simulink model "ThermalMon"  (R2023b)
settings: Solver=FixedStepAuto  StartTime=0.0  StopTime=10.0  RelTol=1e-3
undefined symbols (not defined in the file): THERMALMON_FILTER_ALPHA, THERMALMON_T_CRITICAL_TH, THERMALMON_T_OVERHEAT_TH, THERMALMON_T_UNDER_TH, THERMALMON_T_WARNING_TH, THERMALMON_TS_SEC, ThermalState_e
libraries: simulink x10
settings Model: DataDictionary=ThermalMon.sldd  Creator=84339  LastModifiedBy=84339
settings OptimizationCC: DefaultParameterBehavior=Inlined  EnhancedBackFolding=on  PassReuseOutputArgsAs=Individual arguments  ZeroExternalMemoryAtStartup=off  ZeroInternalMemoryAtStartup=off  OptimizeBlockOrder=speed  DifferentSizesBufferReuse=on  OptimizationCustomize=off  EfficientTunableParamExpr=on
settings DebuggingCC: ParameterTunabilityLossMsg=error
settings ModelReferenceCC: ModelReferenceNumInstancesAllowed=Single
settings SFSimCC: MATLABDynamicMemAlloc=off
settings RTWCC: Description=Embedded Coder  SystemTargetFile=ert.tlc  EmbeddedCoderDictionary=ASW.sldd  GenCodeOnly=on  TemplateMakefile=ert_default_tmf  DataTypeReplacement=CDataTypesFixedWidth
settings CodeAppCC: ForceParamTrailComments=on  IgnoreCustomStorageClasses=off  OperatorAnnotations=on  SimulinkDataObjDesc=on  SFDataObjDesc=on  InsertBlockDesc=on
settings ERTTargetCC: TargetLangStandard=C99 (ISO)  GenerateSampleERTMain=on  InlinedParameterPlacement=NonHierarchical  ERTCustomFileTemplate=example_file_process.tlc  MaxIdInt64=INT64_MAX  MinIdInt64=INT64_MIN  MaxIdUint64=UINT64_MAX  MaxIdInt32=INT32_MAX  MinIdInt32=INT32_MIN  MaxIdUint32=UINT32_MAX  MaxIdInt16=INT16_MAX  MinIdInt16=INT16_MIN  MaxIdUint16=UINT16_MAX  MaxIdInt8=INT8_MAX  MinIdInt8=INT8_MIN  MaxIdUint8=UINT8_MAX

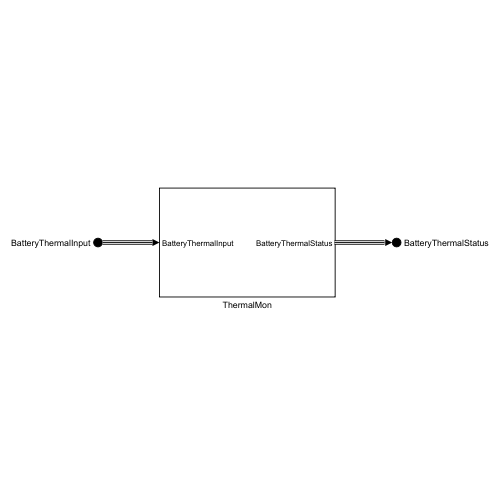
[thumbnail: Simulink's stored preview of the top-level diagram]
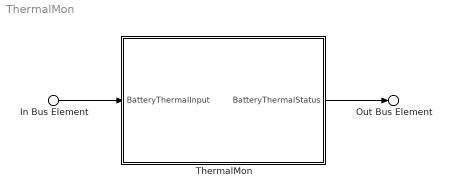
== system ThermalMon ==
  In Bus Element : Inport  PortName=BatteryThermalInput
  ThermalMon : Subsystem
      settings: RTWFcnNameOpts=Use subsystem name
  Out Bus Element : Outport  PortName=BatteryThermalStatus
  wires:
  In Bus Element/1 -> ThermalMon/1(BatteryThermalInput)
  ThermalMon/1(BatteryThermalStatus) -> Out Bus Element/1

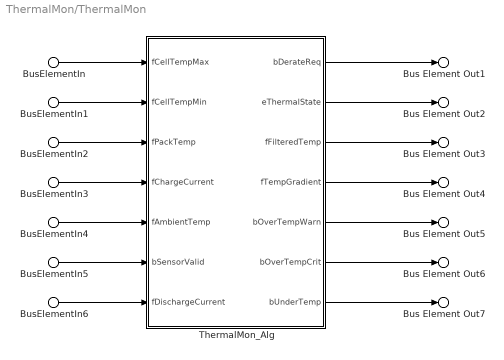
== system ThermalMon/ThermalMon ==
  BusElementIn : Inport  PortName=BatteryThermalInput  Element=fCellTempMax
  BusElementIn1 : Inport  PortName=BatteryThermalInput  Element=fCellTempMin
  BusElementIn2 : Inport  PortName=BatteryThermalInput  Element=fPackTemp
  BusElementIn3 : Inport  PortName=BatteryThermalInput  Element=fChargeCurrent
  BusElementIn4 : Inport  PortName=BatteryThermalInput  Element=fAmbientTemp
  BusElementIn5 : Inport  PortName=BatteryThermalInput  Element=bSensorValid
  BusElementIn6 : Inport  PortName=BatteryThermalInput  Element=fDischargeCurrent
  ThermalMon_Alg : Subsystem
      settings: RTWFcnNameOpts=Use subsystem name
  Bus Element Out2 : Outport  PortName=BatteryThermalStatus  Element=eThermalState
  Bus Element Out3 : Outport  PortName=BatteryThermalStatus  Element=fFilteredTemp
  Bus Element Out4 : Outport  PortName=BatteryThermalStatus  Element=fTempGradient
  Bus Element Out5 : Outport  PortName=BatteryThermalStatus  Element=bOverTempWarn
  Bus Element Out6 : Outport  PortName=BatteryThermalStatus  Element=bOverTempCrit
  Bus Element Out1 : Outport  PortName=BatteryThermalStatus  Element=bDerateReq
  Bus Element Out7 : Outport  PortName=BatteryThermalStatus  Element=bUnderTemp
  wires:
  BusElementIn/1 -> ThermalMon_Alg/1(fCellTempMax)
  BusElementIn1/1 -> ThermalMon_Alg/2(fCellTempMin)
  ThermalMon_Alg/1(bDerateReq) -> Bus Element Out1/1
  ThermalMon_Alg/2(eThermalState) -> Bus Element Out2/1
  ThermalMon_Alg/3(fFilteredTemp) -> Bus Element Out3/1
  ThermalMon_Alg/4(fTempGradient) -> Bus Element Out4/1
  ThermalMon_Alg/5(bOverTempWarn) -> Bus Element Out5/1
  ThermalMon_Alg/6(bOverTempCrit) -> Bus Element Out6/1
  BusElementIn6/1 -> ThermalMon_Alg/7(fDischargeCurrent)
  BusElementIn2/1 -> ThermalMon_Alg/3(fPackTemp)
  BusElementIn3/1 -> ThermalMon_Alg/4(fChargeCurrent)
  BusElementIn4/1 -> ThermalMon_Alg/5(fAmbientTemp)
  BusElementIn5/1 -> ThermalMon_Alg/6(bSensorValid)
  ThermalMon_Alg/7(bUnderTemp) -> Bus Element Out7/1

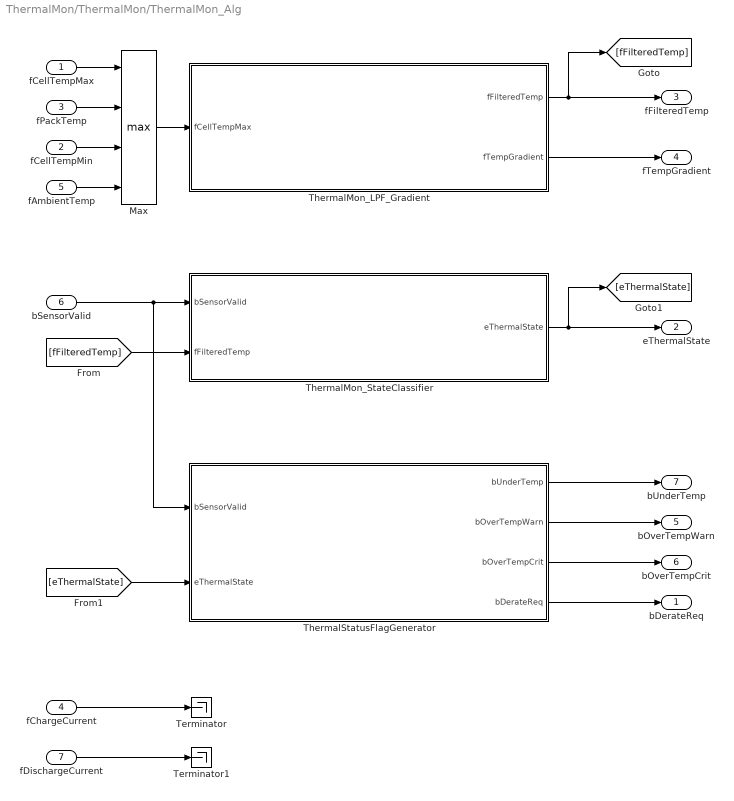
== system ThermalMon/ThermalMon/ThermalMon_Alg ==
  fCellTempMax : Inport  OutDataTypeStr=single
  fCellTempMin : Inport  Port=2  OutDataTypeStr=single
  fPackTemp : Inport  Port=3  OutDataTypeStr=single
  fChargeCurrent : Inport  Port=4  OutDataTypeStr=single
  fAmbientTemp : Inport  Port=5  OutDataTypeStr=single
  bSensorValid : Inport  Port=6  OutDataTypeStr=boolean
  fDischargeCurrent : Inport  Port=7  OutDataTypeStr=single
  Max : MinMax  Function=max  Inputs=4  OutDataTypeStr=single
  Terminator : Terminator
  Terminator1 : Terminator
  ThermalMon_LPF_Gradient : Subsystem  TreatAsAtomicUnit=on
      settings: RTWSystemCode=Nonreusable function  RTWFcnNameOpts=Use subsystem name
  ThermalMon_StateClassifier : Subsystem  TreatAsAtomicUnit=on
      settings: RTWSystemCode=Nonreusable function  RTWFcnNameOpts=Use subsystem name
  ThermalStatusFlagGenerator : Subsystem  TreatAsAtomicUnit=on
      settings: RTWSystemCode=Nonreusable function  RTWFcnNameOpts=Use subsystem name
  bDerateReq : Outport  OutDataTypeStr=boolean
  eThermalState : Outport  Port=2  OutDataTypeStr=Enum: ThermalState_e
  fFilteredTemp : Outport  Port=3  OutDataTypeStr=single
  fTempGradient : Outport  Port=4  OutDataTypeStr=single
  bOverTempWarn : Outport  Port=5  OutDataTypeStr=boolean
  bOverTempCrit : Outport  Port=6  OutDataTypeStr=boolean
  bUnderTemp : Outport  Port=7  OutDataTypeStr=boolean
  wires:
  [fFilteredTemp] -> ThermalMon_StateClassifier/2(fFilteredTemp)
  fPackTemp/1 -> Max/2
  ThermalMon_LPF_Gradient/1(fFilteredTemp) -> fFilteredTemp/1, [fFilteredTemp]
  bSensorValid/1 -> ThermalStatusFlagGenerator/1(bSensorValid), ThermalMon_StateClassifier/1(bSensorValid)
  Max/1 -> ThermalMon_LPF_Gradient/1(fCellTempMax)
  ThermalMon_LPF_Gradient/2(fTempGradient) -> fTempGradient/1
  [eThermalState] -> ThermalStatusFlagGenerator/2(eThermalState)
  fDischargeCurrent/1 -> Terminator1/1
  fChargeCurrent/1 -> Terminator/1
  ThermalStatusFlagGenerator/1(bUnderTemp) -> bUnderTemp/1
  ThermalStatusFlagGenerator/3(bOverTempCrit) -> bOverTempCrit/1
  ThermalStatusFlagGenerator/4(bDerateReq) -> bDerateReq/1
  fCellTempMax/1 -> Max/1
  fCellTempMin/1 -> Max/3
  ThermalMon_StateClassifier/1(eThermalState) -> [eThermalState], eThermalState/1
  fAmbientTemp/1 -> Max/4
  ThermalStatusFlagGenerator/2(bOverTempWarn) -> bOverTempWarn/1

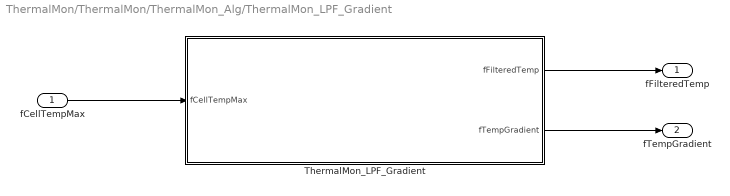
== system ThermalMon/ThermalMon/ThermalMon_Alg/ThermalMon_LPF_Gradient ==
  fCellTempMax : Inport
  ThermalMon_LPF_Gradient : MATLAB Function  TreatAsAtomicUnit=on
  fFilteredTemp : Outport
  fTempGradient : Outport  Port=2
  wires:
  fCellTempMax/1 -> ThermalMon_LPF_Gradient/1(fCellTempMax)
  ThermalMon_LPF_Gradient/1(fFilteredTemp) -> fFilteredTemp/1
  ThermalMon_LPF_Gradient/2(fTempGradient) -> fTempGradient/1

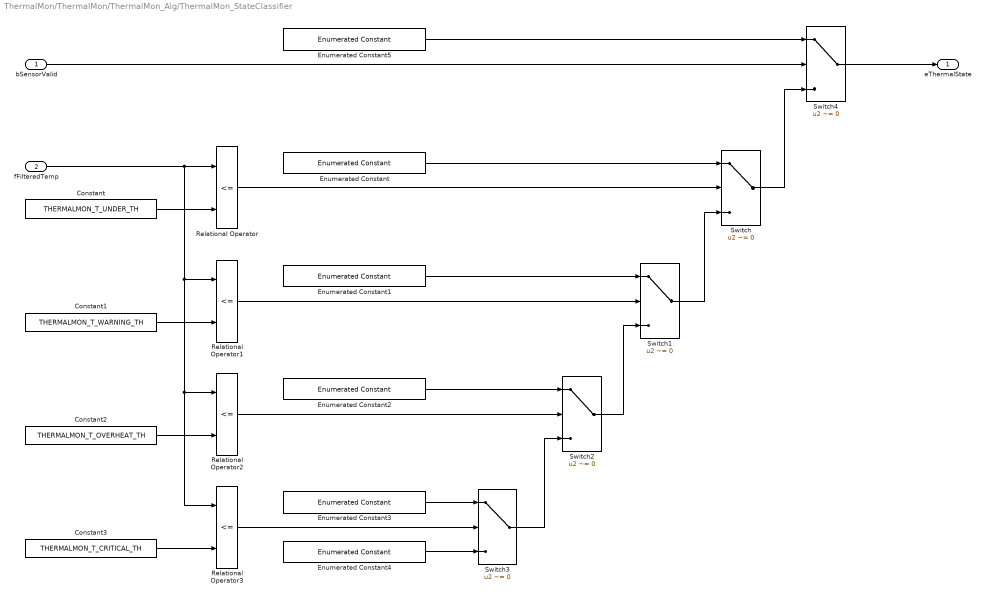
== system ThermalMon/ThermalMon/ThermalMon_Alg/ThermalMon_StateClassifier ==
  bSensorValid : Inport
  fFilteredTemp : Inport  Port=2
  Constant : Constant  Value=THERMALMON_T_UNDER_TH
  Constant1 : Constant  Value=THERMALMON_T_WARNING_TH
  Constant2 : Constant  Value=THERMALMON_T_OVERHEAT_TH
  Constant3 : Constant  Value=THERMALMON_T_CRITICAL_TH
  Enumerated Constant : simulink/Sources/Enumerated Constant  OutDataTypeStr=Enum: ThermalState_e  Value=ThermalState_e.THERM_UNDER_TEMP  SampleTime=inf
  Enumerated Constant1 : simulink/Sources/Enumerated Constant  OutDataTypeStr=Enum: ThermalState_e  Value=ThermalState_e.THERM_NORMAL  SampleTime=inf
  Enumerated Constant2 : simulink/Sources/Enumerated Constant  OutDataTypeStr=Enum: ThermalState_e  Value=ThermalState_e.THERM_WARNING  SampleTime=inf
  Enumerated Constant3 : simulink/Sources/Enumerated Constant  OutDataTypeStr=Enum: ThermalState_e  Value=ThermalState_e.THERM_OVERHEAT  SampleTime=inf
  Enumerated Constant4 : simulink/Sources/Enumerated Constant  OutDataTypeStr=Enum: ThermalState_e  Value=ThermalState_e.THERM_CRITICAL  SampleTime=inf
  Enumerated Constant5 : simulink/Sources/Enumerated Constant  OutDataTypeStr=Enum: ThermalState_e  Value=ThermalState_e.THERM_CRITICAL  SampleTime=inf
  Relational Operator{,1..3} (4 alike) : RelationalOperator  Operator=<=  OutDataTypeStr=boolean  RndMeth=Simplest  InputSameDT=off
  Switch{,1..4} (5 alike) : Switch  Criteria=u2 ~= 0  SaturateOnIntegerOverflow=off  InputSameDT=off
  eThermalState : Outport
  wires:
  Relational Operator/1 -> Switch/2
  Constant/1 -> Relational Operator/2
  Enumerated Constant/1 -> Switch/1
  Relational Operator1/1 -> Switch1/2
  Constant1/1 -> Relational Operator1/2
  Enumerated Constant1/1 -> Switch1/1
  Constant2/1 -> Relational Operator2/2
  Enumerated Constant2/1 -> Switch2/1
  Relational Operator2/1 -> Switch2/2
  Relational Operator3/1 -> Switch3/2
  Enumerated Constant3/1 -> Switch3/1
  Constant3/1 -> Relational Operator3/2
  fFilteredTemp/1 -> Relational Operator/1, Relational Operator1/1, Relational Operator2/1, Relational Operator3/1
  Enumerated Constant4/1 -> Switch3/3
  Switch1/1 -> Switch/3
  Switch3/1 -> Switch2/3
  Switch2/1 -> Switch1/3
  bSensorValid/1 -> Switch4/2
  Enumerated Constant5/1 -> Switch4/1
  Switch/1 -> Switch4/3
  Switch4/1 -> eThermalState/1

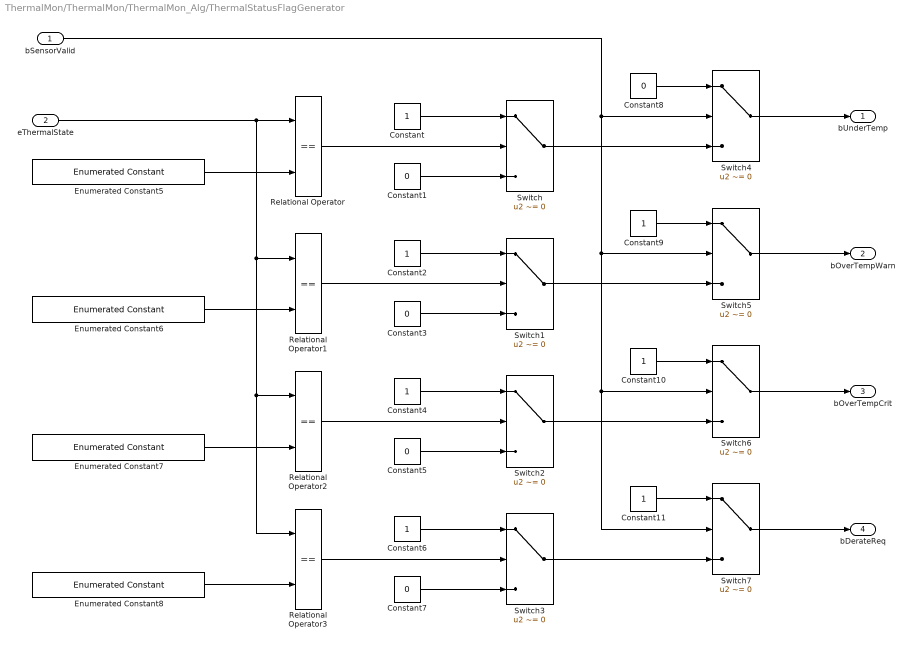
== system ThermalMon/ThermalMon/ThermalMon_Alg/ThermalStatusFlagGenerator ==
  bSensorValid : Inport
  eThermalState : Inport  Port=2
  Constant{,2,4,6,9..11} (7 alike) : Constant  OutDataTypeStr=boolean
  Constant{1,3,5,7..8} (5 alike) : Constant  Value=0  OutDataTypeStr=boolean
  Enumerated Constant5 : simulink/Sources/Enumerated Constant  OutDataTypeStr=Enum: ThermalState_e  Value=ThermalState_e.THERM_UNDER_TEMP  SampleTime=inf
  Enumerated Constant6 : simulink/Sources/Enumerated Constant  OutDataTypeStr=Enum: ThermalState_e  Value=ThermalState_e.THERM_WARNING  SampleTime=inf
  Enumerated Constant7 : simulink/Sources/Enumerated Constant  OutDataTypeStr=Enum: ThermalState_e  Value=ThermalState_e.THERM_OVERHEAT  SampleTime=inf
  Enumerated Constant8 : simulink/Sources/Enumerated Constant  OutDataTypeStr=Enum: ThermalState_e  Value=ThermalState_e.THERM_CRITICAL  SampleTime=inf
  Relational Operator{,1..3} (4 alike) : RelationalOperator  Operator===  OutDataTypeStr=boolean  RndMeth=Simplest  InputSameDT=off
  Switch{,1..7} (8 alike) : Switch  Criteria=u2 ~= 0  SaturateOnIntegerOverflow=off  InputSameDT=off
  bUnderTemp : Outport
  bOverTempWarn : Outport  Port=2
  bOverTempCrit : Outport  Port=3
  bDerateReq : Outport  Port=4
  wires:
  Relational Operator/1 -> Switch/2
  Enumerated Constant5/1 -> Relational Operator/2
  Constant/1 -> Switch/1
  Relational Operator1/1 -> Switch1/2
  Enumerated Constant6/1 -> Relational Operator1/2
  Enumerated Constant7/1 -> Relational Operator2/2
  Enumerated Constant8/1 -> Relational Operator3/2
  eThermalState/1 -> Relational Operator/1, Relational Operator1/1, Relational Operator2/1, Relational Operator3/1
  Constant1/1 -> Switch/3
  Constant3/1 -> Switch1/3
  Constant2/1 -> Switch1/1
  Constant5/1 -> Switch2/3
  Constant4/1 -> Switch2/1
  Constant7/1 -> Switch3/3
  Constant6/1 -> Switch3/1
  Relational Operator3/1 -> Switch3/2
  Relational Operator2/1 -> Switch2/2
  Constant8/1 -> Switch4/1
  Switch/1 -> Switch4/3
  Switch4/1 -> bUnderTemp/1
  Constant9/1 -> Switch5/1
  Switch1/1 -> Switch5/3
  Switch5/1 -> bOverTempWarn/1
  Constant10/1 -> Switch6/1
  Switch2/1 -> Switch6/3
  Switch6/1 -> bOverTempCrit/1
  bSensorValid/1 -> Switch6/2, Switch7/2, Switch5/2, Switch4/2
  Switch7/1 -> bDerateReq/1
  Constant11/1 -> Switch7/1
  Switch3/1 -> Switch7/3

== matlab function ThermalMon/ThermalMon_Alg/ThermalMon_LPF_Gradient/ThermalMon_LPF_Gradient ==
  data: fCellTempMax input; fFilteredTemp output; THERMALMON_FILTER_ALPHA parameter; fTempGradient output; THERMALMON_TS_SEC parameter
function [fFilteredTemp,fTempGradient] = ThermalMon_LPF_Gradient(fCellTempMax, THERMALMON_FILTER_ALPHA, THERMALMON_TS_SEC)
    %#codegen
    % Low-pass filter for battery temperature (ThermalMonitor)
    
    % === Persistent variable (memory) ===
    persistent fFilteredTemp_prev
    if isempty(fFilteredTemp_prev)
        % Initialization at first execution
        fFilteredTemp_prev = fCellTempMax;
    end
    
    % === Low-pass filter equation ===
    % fFilteredTemp(k) = fFilteredTemp(k-1)
    %                 + alpha * (fCellTempMax - fFilteredTemp(k-1))
    fFilteredTemp = fFilteredTemp_prev + THERMALMON_FILTER_ALPHA * (fCellTempMax - fFilteredTemp_prev);
    
    % ===== Temperature gradient =====
    % TempGradient = (FilteredTemp(k) - FilteredTemp(k-1)) / Ts
    fTempGradient = (fFilteredTemp - fFilteredTemp_prev) / THERMALMON_TS_SEC;
    
    % === Update memory ===
    fFilteredTemp_prev = fFilteredTemp;
end
